simulink model "struktura_obserwatora"  (R2023a)
settings: Solver=VariableStepAuto  StartTime=0.0  StopTime=10.0  RelTol=1e-3
values from neighbouring files (symbols this model uses):
  L = acker(A', C', [s0, s0, s0])    [do_workspace.m]    (also in zadania_1_5.m)
settings Model: Creator=adams  LastModifiedBy=adams

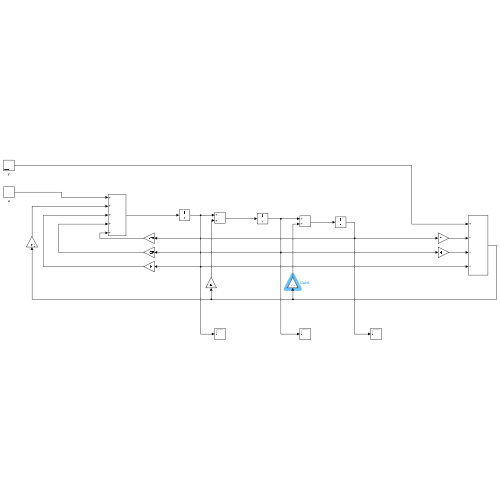
[thumbnail: Simulink's stored preview of the top-level diagram]
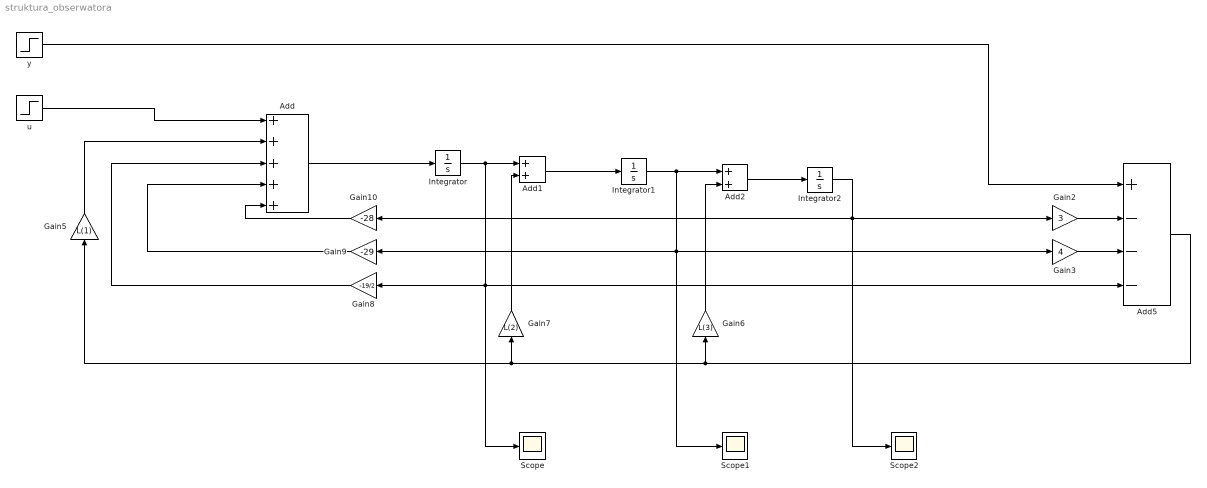
== system struktura_obserwatora ==
  Add : Sum  Inputs=+++++
  Add1 : Sum
  Add2 : Sum
  Add5 : Sum  Inputs=+---
  Gain10 : Gain  Gain=-28
  Gain2 : Gain  Gain=3
  Gain3 : Gain  Gain=4
  Gain5 : Gain  Gain=L(1)
  Gain6 : Gain  Gain=L(3)
  Gain7 : Gain  Gain=L(2)
  Gain8 : Gain  Gain=-19/2
  Gain9 : Gain  Gain=-29
  Integrator : Integrator
  Integrator1 : Integrator
  Integrator2 : Integrator
  Scope : Scope
  Scope1 : Scope
  Scope2 : Scope
  u : Step  SampleTime=0
  y : Step  SampleTime=0
  wires:
  Add1/1 -> Integrator1/1
  Integrator/1 -> Scope/1, Gain8/1, Add5/4, Add1/1
  Add2/1 -> Integrator2/1
  Integrator1/1 -> Scope1/1, Gain9/1, Gain3/1, Add2/1
  Integrator2/1 -> Scope2/1, Gain2/1, Gain10/1
  Gain2/1 -> Add5/2
  Gain3/1 -> Add5/3
  Add5/1 -> Gain7/1, Gain5/1, Gain6/1
  Gain6/1 -> Add2/2
  u/1 -> Add/1
  Add/1 -> Integrator/1
  Gain5/1 -> Add/2
  Gain7/1 -> Add1/2
  Gain8/1 -> Add/3
  Gain9/1 -> Add/4
  Gain10/1 -> Add/5
  y/1 -> Add5/1
